simulink model "Monitor_nounits"  (R2017b)
settings: Solver=VariableStepAuto  StartTime=0.0  StopTime=10.0  RelTol=1e-3
libraries: simulink x1
settings Model: Creator=eh6qym  LastModifiedBy=eh6qym

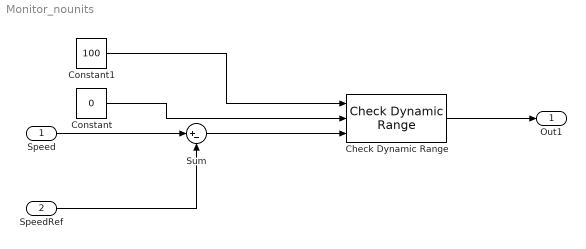
== system Monitor_nounits ==
  Speed : Inport  OutDataTypeStr=double
  SpeedRef : Inport  Port=2  OutDataTypeStr=double
  Check Dynamic Range : simulink/Model Verification/Check  Dynamic Range  Description=min < u < max  enabled=on  stopWhenAssertionFail=on  export=on  icon=graphic
      settings: SourceProductName=Simulink  SourceProductBaseCode=SL
  Constant : Constant  Value=0
  Constant1 : Constant  Value=100
  Sum : Sum  Inputs=|+-
  Out1 : Outport  OutDataTypeStr=boolean
  wires:
  Speed/1 -> Sum/1
  SpeedRef/1 -> Sum/2
  Sum/1 -> Check Dynamic Range/3
  Constant1/1 -> Check Dynamic Range/1
  Constant/1 -> Check Dynamic Range/2
  Check Dynamic Range/1 -> Out1/1
